simulink model "gm_AMdemod_vnl"  (R2021a)
settings: Solver=VariableStepAuto  StartTime=0.0  StopTime=10.0  RelTol=1e-3
libraries: hdlsllib x4, dspsrcs4 x3, simulink x2
settings Model: Creator=guido  LastModifiedBy=guido
settings OptimizationCC: BlockReduction=off  ConditionallyExecuteInputs=off  DefaultParameterBehavior=Inlined
settings DebuggingCC: AlgebraicLoopMsg=error  InheritedTsInSrcMsg=none
settings HardwareCC: ProdBitPerPointer=32  ProdBitPerSizeT=32  ProdBitPerPtrDiffT=32  ProdLargestAtomicFloat=None  ProdIntDivRoundTo=Undefined  ProdEndianess=Unspecified  ProdWordSize=32  ProdHWDeviceType=ASIC/FPGA->ASIC/FPGA  TargetBitPerPointer=64  TargetBitPerSizeT=64  TargetBitPerPtrDiffT=64  TargetLongLongMode=on  TargetIntDivRoundTo=Zero  TargetEndianess=LittleEndian  TargetWordSize=64  TargetHWDeviceType=Custom Processor->MATLAB Host Computer  ProdEqTarget=off

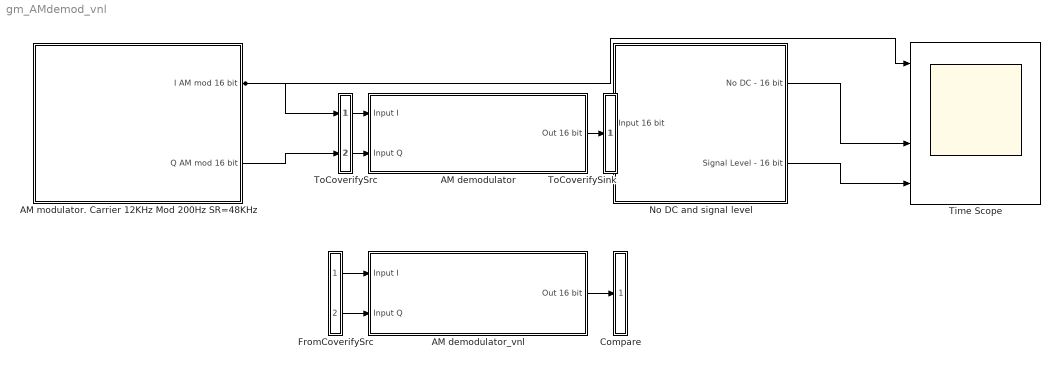
== system gm_AMdemod_vnl ==
  AM demodulator : Subsystem
  AM demodulator_vnl : Subsystem
  "AM modulator. Carrier 12KHz Mod 200Hz SR=48KHz " : Subsystem
  Compare : Subsystem
      mask Display: disp('')
  FromCoverifySrc : Subsystem
      mask Display: disp('')
  No DC and signal level : Subsystem
  Time Scope : Scope  NumInputPorts=4
  ToCoverifySink : Subsystem
      mask Display: disp('')
  ToCoverifySrc : Subsystem
      mask Display: disp('')
  wires:
  No DC and signal level/2("Signal Level - 16 bit ") -> Time Scope/4
  No DC and signal level/1(No DC - 16 bit) -> Time Scope/3
  "AM modulator. Carrier 12KHz Mod 200Hz SR=48KHz "/1(I AM mod 16 bit) -> Time Scope/1, ToCoverifySrc/1(in1)
  ToCoverifySrc/1(out1) -> AM demodulator/1(Input I)
  ToCoverifySrc/2(out2) -> AM demodulator/2(Input Q)
  AM demodulator/1(Out 16 bit) -> ToCoverifySink/1(in1)
  "AM modulator. Carrier 12KHz Mod 200Hz SR=48KHz "/2(Q AM mod 16 bit) -> ToCoverifySrc/2(in2)
  ToCoverifySink/1(out1) -> No DC and signal level/1(Input 16 bit)
  FromCoverifySrc/1(out1) -> AM demodulator_vnl/1(Input I)
  FromCoverifySrc/2(out2) -> AM demodulator_vnl/2(Input Q)
  AM demodulator_vnl/1(Out 16 bit) -> Compare/1(in1)

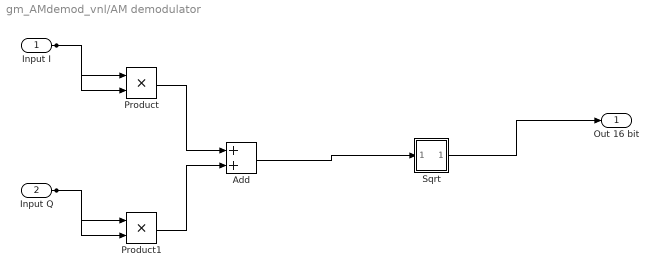
== system gm_AMdemod_vnl/AM demodulator ==
  Input I : Inport  OutDataTypeStr=int32  PortDimensions=1  SampleTime=1e-09
  Input Q : Inport  Port=2  OutDataTypeStr=int32  PortDimensions=1  SampleTime=1e-09
  Add : Sum  AccumDataTypeStr=fixdt(1, 65, 0)  OutDataTypeStr=fixdt(1, 65, 0)  SampleTime=1e-09
  Product : Product  Inputs=**  OutDataTypeStr=fixdt(1, 64, 0)  SampleTime=1e-09
  Product1 : Product  Inputs=**  OutDataTypeStr=fixdt(1, 64, 0)  SampleTime=1e-09
  Sqrt : Subsystem
  Out 16 bit : Outport  SampleTime=1e-09
  wires:
  Sqrt/1(Out1) -> Out 16 bit/1
  Product1/1 -> Add/2
  Product/1 -> Add/1
  Add/1 -> Sqrt/1(In1)
  Input Q/1 -> Product1/1, Product1/2
  Input I/1 -> Product/1, Product/2

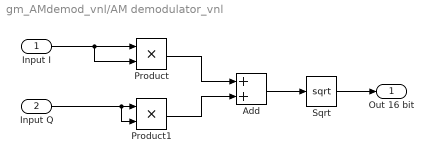
== system gm_AMdemod_vnl/AM demodulator_vnl ==
  Input I : Inport  SampleTime=10^-9
  Input Q : Inport  Port=2  SampleTime=10^-9
  Add : Sum
  Product : Product
  Product1 : Product
  Sqrt : Sqrt  OutDataTypeStr=int16  SaturateOnIntegerOverflow=on
  Out 16 bit : Outport
  wires:
  Sqrt/1 -> Out 16 bit/1
  Input Q/1 -> Product1/1, Product1/2
  Input I/1 -> Product/2, Product/1
  Product/1 -> Add/1
  Add/1 -> Sqrt/1
  Product1/1 -> Add/2

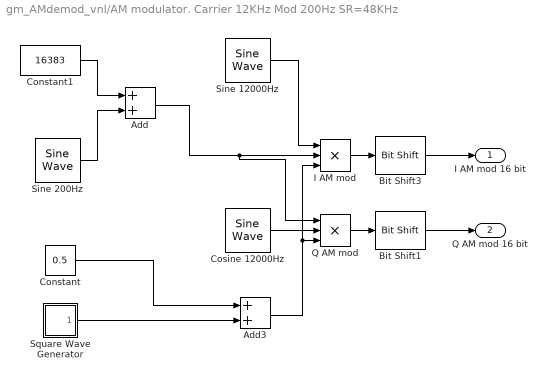
== system gm_AMdemod_vnl/AM modulator. Carrier 12KHz Mod 200Hz SR=48KHz  ==
  Add : Sum  AccumDataTypeStr=int16  OutDataTypeStr=int16
  Add3 : Sum
  Bit Shift1 : hdlsllib/Logic and Bit Operations/Bit Shift  mode=Shift Right Arithmetic  N=16
  Bit Shift3 : hdlsllib/Logic and Bit Operations/Bit Shift  mode=Shift Right Arithmetic  N=16
  Constant : Constant  Value=0.5
  Constant1 : Constant  Value=16383  OutDataTypeStr=int16
  Cosine 12000Hz : dspsrcs4/Sine Wave  Amplitude=32767  Frequency=12000  Phase=pi/2  SampleMode=Discrete  OutComplex=Real  CompMethod=Table lookup  TableSize=Speed  SampleTime=1/48000  SamplesPerFrame=1  ResetState=Restart at time zero  OutputFrames=off  dataType=Fixed-point  wordLen=16  udDataType=sfix(16)  fracBitsMode=Best precision  numFracBits=0  OutDataTypeStr=fixdt(1,16)  LastOutDataTypeStr=fixdt(1,16)
  I AM mod : Product  Inputs=3  OutDataTypeStr=int32  SaturateOnIntegerOverflow=on
  Q AM mod : Product  Inputs=3  OutDataTypeStr=int32  SaturateOnIntegerOverflow=on
  Sine 12000Hz : dspsrcs4/Sine Wave  Amplitude=32767  Frequency=12000  Phase=0  SampleMode=Discrete  OutComplex=Real  CompMethod=Table lookup  TableSize=Speed  SampleTime=1/48000  SamplesPerFrame=1  ResetState=Restart at time zero  OutputFrames=off  dataType=Fixed-point  wordLen=16  udDataType=sfix(16)  fracBitsMode=Best precision  numFracBits=0  OutDataTypeStr=fixdt(1,16)  LastOutDataTypeStr=fixdt(1,16)
  Sine 200Hz : dspsrcs4/Sine Wave  Amplitude=16000  Frequency=800  Phase=0  SampleMode=Discrete  OutComplex=Real  CompMethod=Table lookup  TableSize=Speed  SampleTime=1/48000  SamplesPerFrame=1  ResetState=Restart at time zero  OutputFrames=off  dataType=Fixed-point  wordLen=16  udDataType=sfix(16)  fracBitsMode=Best precision  numFracBits=0  OutDataTypeStr=fixdt(1,16)  LastOutDataTypeStr=fixdt(1,16)
  Square Wave Generator : Subsystem  Tag=DecoupledSystem
  I AM mod 16 bit : Outport
  Q AM mod 16 bit : Outport  Port=2
  wires:
  Add3/1 -> I AM mod/3, Q AM mod/3
  Sine 12000Hz/1 -> I AM mod/1
  Add/1 -> Q AM mod/1, I AM mod/2
  Cosine 12000Hz/1 -> Q AM mod/2
  Constant/1 -> Add3/1
  Sine 200Hz/1 -> Add/2
  Square Wave Generator/1(Out1) -> Add3/2
  Constant1/1 -> Add/1
  I AM mod/1 -> Bit Shift3/1
  Q AM mod/1 -> Bit Shift1/1
  Bit Shift3/1 -> I AM mod 16 bit/1
  Bit Shift1/1 -> Q AM mod 16 bit/1

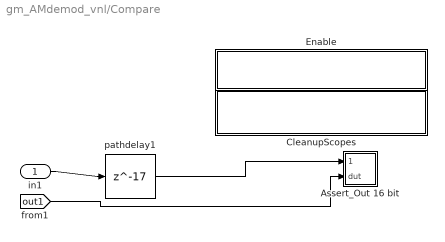
== system gm_AMdemod_vnl/Compare ==
  in1 : Inport
  Assert_Out 16 bit : Subsystem
  CleanupScopes : Subsystem
      settings: OpenFcn=|
      | blkName = gcb; %self block
      | idx = regexp(blkName, '/CleanupScopes$', 'once');
      | blkParent = blkName(1:idx-1);
      | blks=find_system(blkParent, 'LookUnderMasks', 'all','blocktype', 'Scope');
      | for itr = 1:length(blks)
      | 	 hScopeCfg = get_param(blks{itr},'ScopeConfiguration');
      | 	 hScopeCfg.Visible = ~ hScopeCfg.Visible;
      | end
      | drawnow;
      mask Display: fprintf(message('hdlcoder:cosim:vnl_dblclick').getString());
  Enable : Subsystem
      settings: OpenFcn=|
      | blkName = gcb;
      | idx = regexp(blkName, '/Enable$', 'once');
      | blkParent = blkName(1:idx-1);
      | blks=find_system(blkParent, 'LookUnderMasks', 'all','blocktype', 'Assertion');
      | e = get_param(blks{1}, 'Enabled');
      | if strcmp(e, 'on'), f= 'off';, else, f = 'on';, end
      | for ii=1:length(blks), set_param(blks{ii}, 'Enabled', f);, end
      | set_param(gcb, 'MaskDisplay',['fprintf(message(''hdlcoder:cosim:vnl_dblclick_assertions'',','''',upper(e),'''',').getString())']);
      mask Display: fprintf(message('hdlcoder:cosim:vnl_dblclick_assertions','OFF').getString());
  pathdelay1 : Delay  DelayLength=17
  wires:
  in1/1 -> pathdelay1/1
  pathdelay1/1 -> Assert_Out 16 bit/1(cosim)
  [out1] -> Assert_Out 16 bit/2(dut)

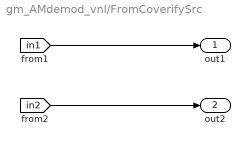
== system gm_AMdemod_vnl/FromCoverifySrc ==
  out1 : Outport
  out2 : Outport  Port=2
  wires:
  [in1] -> out1/1
  [in2] -> out2/1

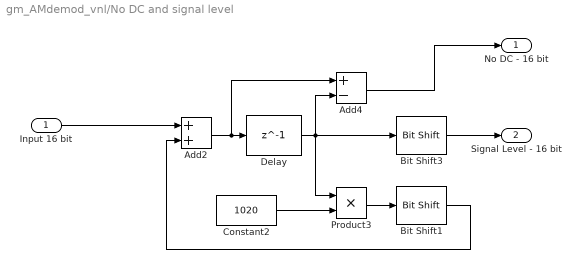
== system gm_AMdemod_vnl/No DC and signal level ==
  Input 16 bit : Inport
  Add2 : Sum  AccumDataTypeStr=int64  OutDataTypeStr=int64
  Add4 : Sum  Inputs=+-  AccumDataTypeStr=int32  OutDataTypeStr=int16
  Bit Shift1 : hdlsllib/Logic and Bit Operations/Bit Shift  mode=Shift Right Arithmetic  N=10
  Bit Shift3 : hdlsllib/Logic and Bit Operations/Bit Shift  mode=Shift Right Arithmetic  N=9
  Constant2 : Constant  Value=1020  OutDataTypeStr=int32
  Delay : Delay  DelayLength=1  InitialCondition=1  UseCircularBuffer=on
  Product3 : Product  OutDataTypeStr=int64
  No DC - 16 bit : Outport
  "Signal Level - 16 bit " : Outport  Port=2
  wires:
  Delay/1 -> Product3/1, Bit Shift3/1, Add4/2
  Constant2/1 -> Product3/2
  Input 16 bit/1 -> Add2/1
  Add2/1 -> Add4/1, Delay/1
  Bit Shift1/1 -> Add2/2
  Bit Shift3/1 -> "Signal Level - 16 bit "/1
  Product3/1 -> Bit Shift1/1
  Add4/1 -> No DC - 16 bit/1

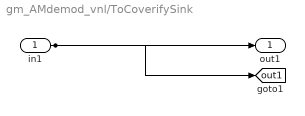
== system gm_AMdemod_vnl/ToCoverifySink ==
  in1 : Inport
  out1 : Outport
  tag scope: out1=global
  wires:
  in1/1 -> out1/1, [out1]

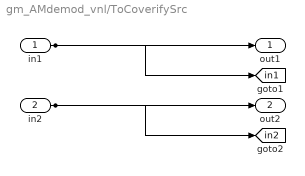
== system gm_AMdemod_vnl/ToCoverifySrc ==
  in1 : Inport
  in2 : Inport  Port=2
  out1 : Outport
  out2 : Outport  Port=2
  tag scope: in1=global, in2=global
  wires:
  in1/1 -> out1/1, [in1]
  in2/1 -> out2/1, [in2]

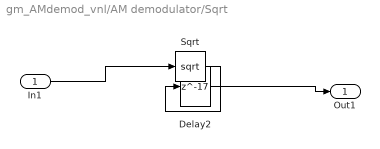
== system gm_AMdemod_vnl/AM demodulator/Sqrt ==
  In1 : Inport
  Delay2 : Delay  DelayLength=17
  Sqrt : Sqrt  OutDataTypeStr=int16  SaturateOnIntegerOverflow=on
  Out1 : Outport
  wires:
  Delay2/1 -> Out1/1
  Sqrt/1 -> Delay2/1
  In1/1 -> Sqrt/1

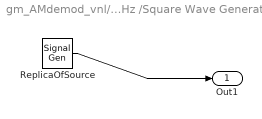
== system gm_AMdemod_vnl/AM modulator. Carrier 12KHz Mod 200Hz SR=48KHz /Square Wave Generator ==
  ReplicaOfSource : SignalGenerator  WaveForm=square  Amplitude=0.5  Frequency=0.5
  Out1 : Outport  LockScale=on
  wires:
  ReplicaOfSource/1 -> Out1/1

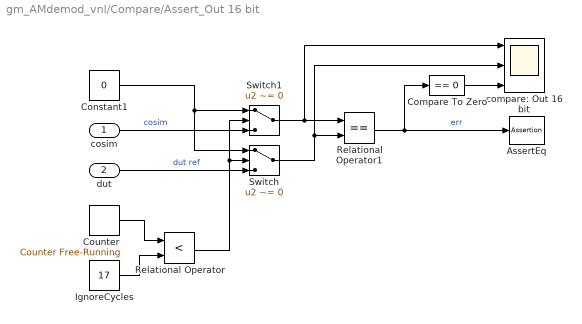
== system gm_AMdemod_vnl/Compare/Assert_Out 16 bit ==
  cosim : Inport
  dut : Inport  Port=2
  AssertEq : Assertion  StopWhenAssertionFail=off
  Compare To Zero : simulink/Logic and Bit Operations/Compare To Zero  relop===  OutDataTypeStr=boolean
  Constant1 : Constant  Value=0  OutDataTypeStr=Inherit: Inherit via back propagation  SampleTime=-1
  Counter : simulink/Sources/Counter Free-Running  NumBits=32  tsamp=-1
  IgnoreCycles : Constant  Value=17  OutDataTypeStr=Inherit: Inherit via back propagation  SampleTime=-1
  Relational Operator : RelationalOperator  Operator=<  OutDataTypeStr=boolean  RndMeth=Nearest
  Relational Operator1 : RelationalOperator  Operator===  OutDataTypeStr=boolean  RndMeth=Nearest
  Switch : Switch  Criteria=u2 ~= 0
  Switch1 : Switch  Criteria=u2 ~= 0
  compare: Out 16 bit : Scope  NumInputPorts=3
  wires:
  Compare To Zero/1 -> compare: Out 16 bit/3
  Relational Operator1/1 -> Compare To Zero/1, AssertEq/1  "err"
  Switch1/1 -> compare: Out 16 bit/1, Relational Operator1/1
  Switch/1 -> compare: Out 16 bit/2, Relational Operator1/2
  Constant1/1 -> Switch/1, Switch1/1
  Relational Operator/1 -> Switch/2, Switch1/2
  cosim/1 -> Switch1/3  "cosim"
  dut/1 -> Switch/3  "dut ref"
  Counter/1 -> Relational Operator/1
  IgnoreCycles/1 -> Relational Operator/2

== system gm_AMdemod_vnl/Compare/CleanupScopes ==

== system gm_AMdemod_vnl/Compare/Enable ==
